simulink model "zad9_2_simulink"  (R2023a)
settings: Solver=VariableStepAuto  StartTime=0.0  StopTime=20  RelTol=1e-3
values from neighbouring files (symbols this model uses):
  Gz = c2d(Gs,T,'zoh')    [zad1.m]
  Kvar_2 = acker(A_var_2,B_var_2,bieguny)    [zad9_nowe_K.m]
  L_np_rz = acker(A_22', A_12', [b_obsv_np_rz, b_obsv_np_rz])'    [zad91.m]
  T = 0.5    [zad1.m]    (also in zad4.mat)
  u_multiply = B_2 - L_np_rz*B_1    [zad91.m]
  w_multiply = (A_22 - L_np_rz*A_12)    [zad91.m]
  y_multiply = A_21 - L_np_rz*A_11    [zad91.m]
settings Model: Creator=pkutyl  LastModifiedBy=pkutyl

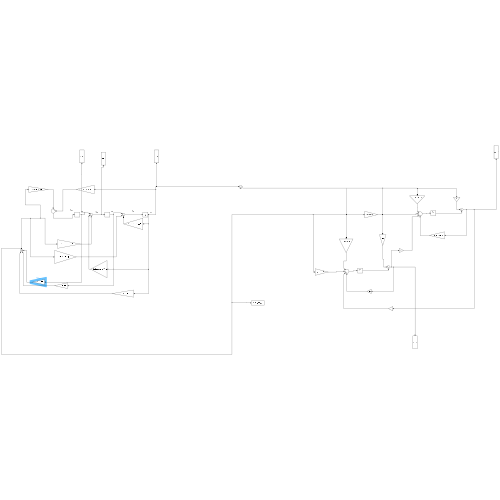
[thumbnail: Simulink's stored preview of the top-level diagram]
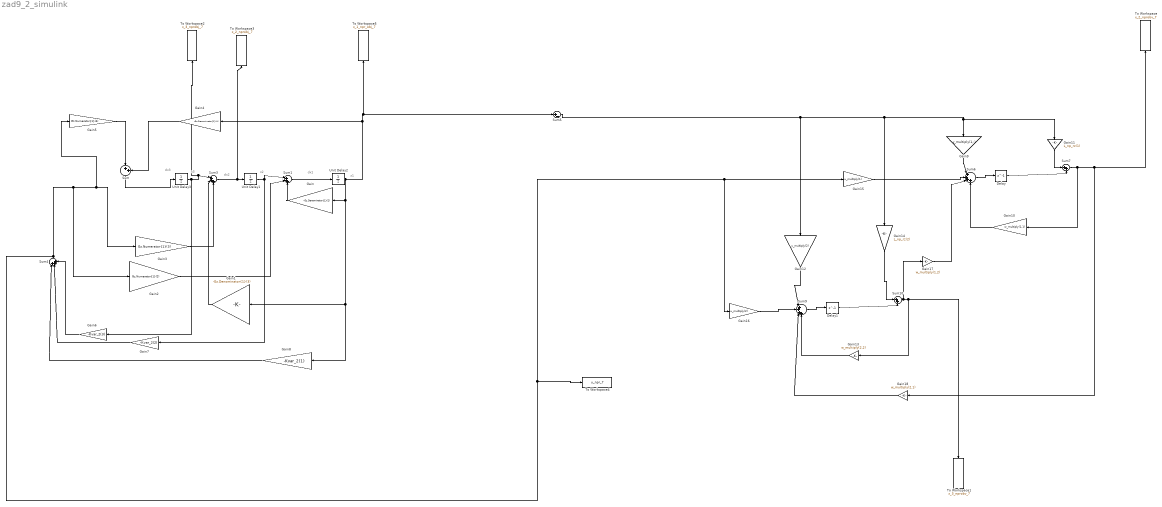
== system zad9_2_simulink ==
  note: x2
  note: dx2
  note: x1
  note: dx1
  note: dx3
  note: x3
  Delay : Delay  DelayLength=1  InitialCondition=0
  Delay1 : Delay  DelayLength=1  InitialCondition=0
  Gain : Gain  Gain=-Gz.Denominator{1}(2)
  Gain1 : Gain  Gain=-Gz.Denominator{1}(3)
  Gain10 : Gain  Gain=w_multiply(1,1)
  Gain11 : Gain  Gain=L_np_rz(1)
  Gain12 : Gain  Gain=y_multiply(2)
  Gain13 : Gain  Gain=w_multiply(2,2)
  Gain14 : Gain  Gain=L_np_rz(2)
  Gain15 : Gain  Gain=u_multiply(1)
  Gain16 : Gain  Gain=u_multiply(2)
  Gain17 : Gain  Gain=w_multiply(1,2)
  Gain18 : Gain  Gain=w_multiply(2,1)
  Gain2 : Gain  Gain=Gz.Numerator{1}(2)
  Gain3 : Gain  Gain=Gz.Numerator{1}(3)
  Gain4 : Gain  Gain=-Gz.Denominator{1}(4)
  Gain5 : Gain  Gain=Gz.Numerator{1}(4)
  Gain6 : Gain  Gain=-Kvar_2(3)
  Gain7 : Gain  Gain=-Kvar_2(2)
  Gain8 : Gain  Gain=-Kvar_2(1)
  Gain9 : Gain  Gain=y_multiply(1,:)
  Sum : Sum  Inputs=|++
  Sum1 : Sum  Inputs=|+++
  Sum10 : Sum  Inputs=|++
  Sum3 : Sum  Inputs=|+++
  Sum4 : Sum  Inputs=|+++
  Sum5 : Sum  Inputs=|+-
  Sum6 : Sum  Inputs=|++++
  Sum7 : Sum  Inputs=|++
  Sum9 : Sum  Inputs=|++++
  To Workspace : ToWorkspace  VariableName=x_2_nprobv_7  SaveFormat=Structure With Time  SampleTime=-1
  To Workspace1 : ToWorkspace  VariableName=x_3_nprobv_7  SaveFormat=Structure With Time  SampleTime=-1
  To Workspace2 : ToWorkspace  VariableName=x_3_nprobj_7  SaveFormat=Structure With Time  SampleTime=-1
  To Workspace3 : ToWorkspace  VariableName=x_2_nprobj_7  SaveFormat=Structure With Time  SampleTime=-1
  To Workspace4 : ToWorkspace  VariableName=u_npr_7  SaveFormat=Structure With Time  SampleTime=-1
  To Workspace5 : ToWorkspace  VariableName=x_1_npr_obj_7  SaveFormat=Structure With Time  SampleTime=-1
  Unit Delay1 : UnitDelay  InitialCondition=1  SampleTime=T  HasFrameUpgradeWarning=on
  Unit Delay2 : UnitDelay  InitialCondition=2  SampleTime=T  HasFrameUpgradeWarning=on
  Unit Delay3 : UnitDelay  InitialCondition=-1  SampleTime=T  HasFrameUpgradeWarning=on
  wires:
  Gain2/1 -> Sum1/2
  Unit Delay2/1 -> Gain4/1, To Workspace5/1, Sum5/1, Gain8/1, Gain1/1, Gain/1
  Gain3/1 -> Sum3/3
  Unit Delay1/1 -> Gain7/1, Sum1/1
  Gain5/1 -> Sum/1
  Gain1/1 -> Sum3/2
  Gain/1 -> Sum1/3
  Gain4/1 -> Sum/2
  Sum1/1 -> Unit Delay2/1
  Sum/1 -> Unit Delay3/1
  Unit Delay3/1 -> Gain6/1, To Workspace2/1, Sum3/1
  Sum3/1 -> Unit Delay1/1, To Workspace3/1
  Gain8/1 -> Sum4/1
  Gain6/1 -> Sum4/3
  Gain7/1 -> Sum4/2
  Sum9/1 -> Delay1/1
  Sum6/1 -> Delay/1
  Gain12/1 -> Sum9/1
  Gain16/1 -> Sum9/2
  Gain11/1 -> Sum7/1
  Gain14/1 -> Sum10/1
  Sum4/1 -> Gain3/1, Gain5/1, Gain2/1, To Workspace4/1, Gain16/1, Gain15/1
  Gain18/1 -> Sum9/3
  Sum10/1 -> Gain17/1, To Workspace1/1, Gain13/1
  Gain13/1 -> Sum9/4
  Gain9/1 -> Sum6/1
  Delay1/1 -> Sum10/2
  Sum5/1 -> Gain11/1, Gain9/1, Gain14/1, Gain12/1
  Sum7/1 -> To Workspace/1, Gain18/1, Gain10/1
  Gain10/1 -> Sum6/4
  Delay/1 -> Sum7/2
  Gain17/1 -> Sum6/3
  Gain15/1 -> Sum6/2
